simulink model "Second_Order_Sytsem_PI_Controller_Series_Parellel_Ideal"  (R2024b)
settings: Solver=VariableStepAuto  StartTime=0.0  StopTime=10.0  RelTol=1e-3
settings Model: Creator=Ahmad  LastModifiedBy=Ahmad

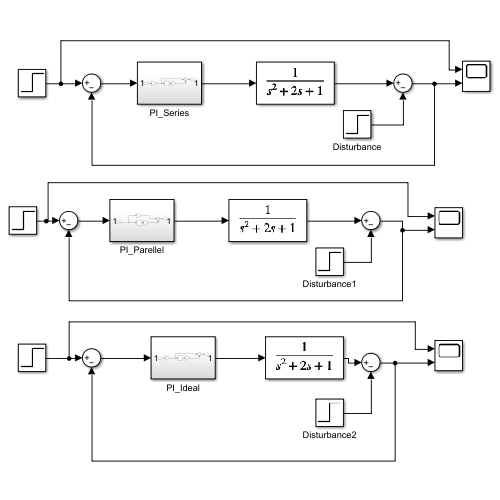
[thumbnail: Simulink's stored preview of the top-level diagram]
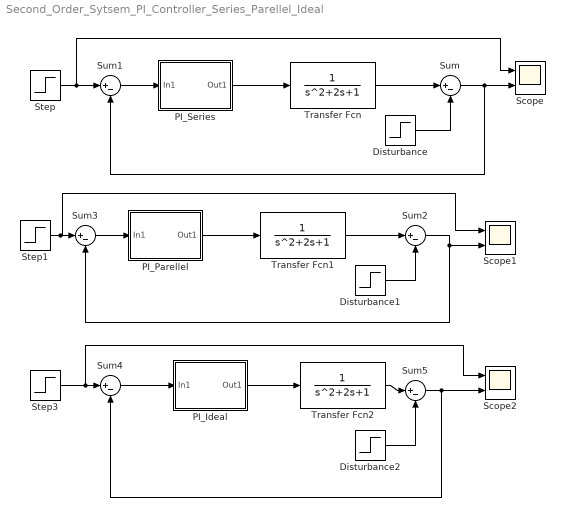
== system Second_Order_Sytsem_PI_Controller_Series_Parellel_Ideal ==
  Disturbance : Step  After=0.5  SampleTime=0
  Disturbance1 : Step  After=0.5  SampleTime=0
  Disturbance2 : Step  After=0.5  SampleTime=0
  PI_Ideal : Subsystem
  PI_Parellel : Subsystem
  PI_Series : Subsystem
  Scope : Scope  NumInputPorts=2
  Scope1 : Scope  NumInputPorts=2
  Scope2 : Scope  NumInputPorts=2
  Step : Step  SampleTime=0
  Step1 : Step  SampleTime=0
  Step3 : Step  SampleTime=0
  Sum{,1..5} (6 alike) : Sum  Inputs=|+-
  Transfer Fcn : TransferFcn
  Transfer Fcn1 : TransferFcn
  Transfer Fcn2 : TransferFcn
  wires:
  Disturbance/1 -> Sum/2
  Transfer Fcn/1 -> Sum/1
  Sum/1 -> Sum1/2, Scope/2
  Step/1 -> Scope/1, Sum1/1
  Sum1/1 -> PI_Series/1(In1)
  PI_Series/1(Out1) -> Transfer Fcn/1
  Transfer Fcn1/1 -> Sum2/1
  Disturbance1/1 -> Sum2/2
  Sum2/1 -> Scope1/2, Sum3/2
  PI_Parellel/1(Out1) -> Transfer Fcn1/1
  Sum3/1 -> PI_Parellel/1(In1)
  Step1/1 -> Scope1/1, Sum3/1
  Step3/1 -> Sum4/1, Scope2/1
  Sum4/1 -> PI_Ideal/1(In1)
  PI_Ideal/1(Out1) -> Transfer Fcn2/1
  Transfer Fcn2/1 -> Sum5/1
  Disturbance2/1 -> Sum5/2
  Sum5/1 -> Sum4/2, Scope2/2

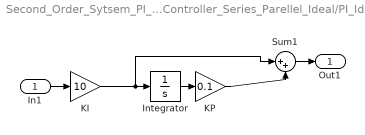
== system Second_Order_Sytsem_PI_Controller_Series_Parellel_Ideal/PI_Ideal ==
  In1 : Inport
  Integrator : Integrator
  KI : Gain  Gain=10
  KP : Gain  Gain=0.1
  Sum1 : Sum  Inputs=|++
  Out1 : Outport
  wires:
  KI/1 -> Sum1/1, Integrator/1
  Integrator/1 -> KP/1
  In1/1 -> KI/1
  KP/1 -> Sum1/2
  Sum1/1 -> Out1/1

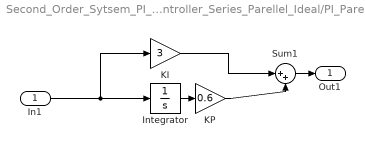
== system Second_Order_Sytsem_PI_Controller_Series_Parellel_Ideal/PI_Parellel ==
  In1 : Inport
  Integrator : Integrator
  KI : Gain  Gain=3
  KP : Gain  Gain=0.6
  Sum1 : Sum  Inputs=|++
  Out1 : Outport
  wires:
  In1/1 -> Integrator/1, KI/1
  Integrator/1 -> KP/1
  KP/1 -> Sum1/2
  Sum1/1 -> Out1/1
  KI/1 -> Sum1/1

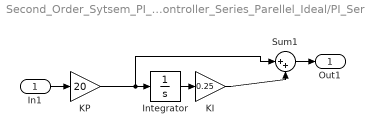
== system Second_Order_Sytsem_PI_Controller_Series_Parellel_Ideal/PI_Series ==
  In1 : Inport
  Integrator : Integrator
  KI : Gain  Gain=0.25
  KP : Gain  Gain=20
  Sum1 : Sum  Inputs=|++
  Out1 : Outport
  wires:
  KP/1 -> Sum1/1, Integrator/1
  Integrator/1 -> KI/1
  In1/1 -> KP/1
  KI/1 -> Sum1/2
  Sum1/1 -> Out1/1
